simulink model "Final_lateral__"  (R2021a)
settings: Solver=VariableStepAuto  StartTime=0.0  StopTime=20  RelTol=1e-3
values from neighbouring files (symbols this model uses):
  A = [-2.3817 0 -1.0019 2.1827; -21.063 -16.055 0.87229 0; 24.512 -16.651 -3.5379 0; 0 1.0026 -0.029766 0]    [lateral_parameters.m]
  B = [0 -0.24719; -36.263 -688.44; -0.6725 -67.983; 0 0]    [lateral_parameters.m]
  B1 = [0.0869 0;4.424 1.184; 0 -1; -2.148 0.021]    [lateral_parameters.m]
  K = [K_hat(:,1) K_hat(:,2) K_hat(:,3) K_hat(:,4)]    [lateral_parameters.m]
  ki = [K_hat(:,5) K_hat(:,6)]    [lateral_parameters.m]
libraries: dspsrcs4 x1
settings Model: Creator=Lenovo  LastModifiedBy=Lenovo

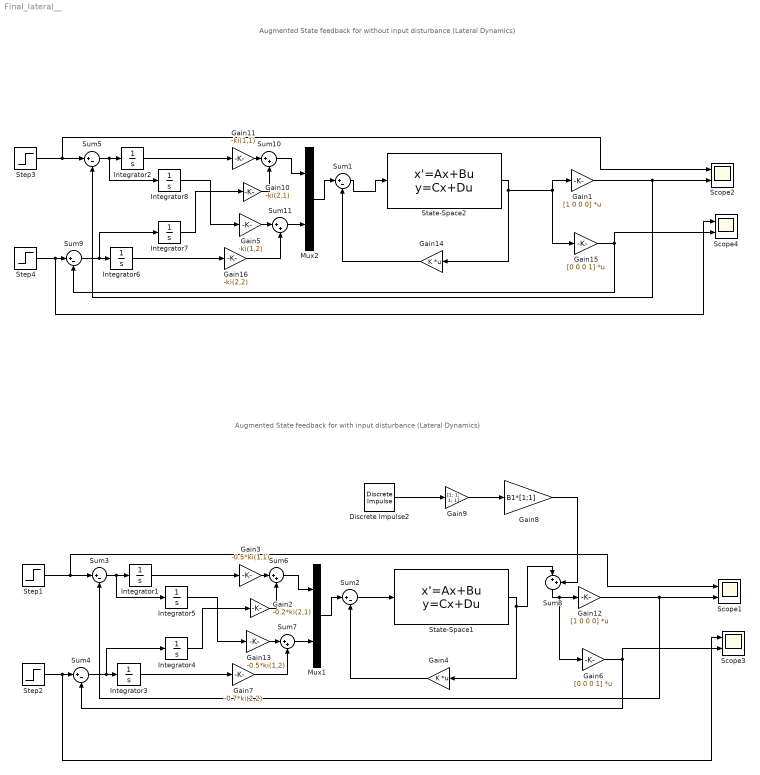
== system Final_lateral__ ==
  note: Augmented State feedback for without input disturbance (Lateral Dynamics)
  note: Augmented State feedback for with input disturbance (Lateral Dynamics)
  Discrete Impulse2 : dspsrcs4/Discrete  Impulse  Delay=0  SampleTime=1  FrameSample=1  OutputFrames=off  dataType=double  isSigned=on  wordLen=16  udDataType=sfix(16)  fracBitsMode=Best precision  numFracBits=15  OutDataTypeStr=double  LastOutDataTypeStr=double
  Gain1 : Gain  Gain=[1 0 0 0]  Multiplication=Matrix(K*u) (u vector)
  Gain10 : Gain  Gain=-ki(2,1)
  Gain11 : Gain  Gain=-ki(1,1)
  Gain12 : Gain  Gain=[1 0 0 0]  Multiplication=Matrix(K*u) (u vector)
  Gain13 : Gain  Gain=-0.5*ki(1,2)
  Gain14 : Gain  Gain=K  Multiplication=Matrix(K*u)
  Gain15 : Gain  Gain=[0 0 0 1]  Multiplication=Matrix(K*u) (u vector)
  Gain16 : Gain  Gain=-ki(2,2)
  Gain2 : Gain  Gain=-0.2*ki(2,1)
  Gain3 : Gain  Gain=-0.5*ki(1,1)
  Gain4 : Gain  Gain=K  Multiplication=Matrix(K*u)
  Gain5 : Gain  Gain=-ki(1,2)
  Gain6 : Gain  Gain=[0 0 0 1]  Multiplication=Matrix(K*u) (u vector)
  Gain7 : Gain  Gain=-0.7*ki(2,2)
  Gain8 : Gain  Gain=B1*[1;1]
  Gain9 : Gain  Gain=[1; 1; 1; 1]
  Integrator{1..8} (8 alike) : Integrator
  Mux1 : Mux  Inputs=2
  Mux2 : Mux  Inputs=2
  Scope{1..4} (4 alike) : Scope  NumInputPorts=2
  State-Space1 : StateSpace  A=A  B=B  C=eye(4)  D=zeros(4,2)  InitialCondition=0
  State-Space2 : StateSpace  A=A  B=B  C=eye(4)  D=zeros(4,2)  InitialCondition=0
  Step{1..4} (4 alike) : Step  Time=0  After=0.2  SampleTime=0
  Sum{1..5,9} (6 alike) : Sum  Inputs=|+-
  Sum{6..8,10..11} (5 alike) : Sum  Inputs=|++
  wires:
  Gain9/1 -> Gain8/1
  Discrete Impulse2/1 -> Gain9/1
  Sum2/1 -> State-Space1/1
  Integrator3/1 -> Gain7/1
  Gain6/1 -> Scope3/2, Sum4/2
  Sum3/1 -> Integrator5/1, Integrator1/1
  Step2/1 -> Scope3/1, Sum4/1
  Step1/1 -> Sum3/1, Scope1/1
  State-Space1/1 -> Sum8/1, Gain4/1
  Gain12/1 -> Scope1/2, Sum3/2
  Integrator1/1 -> Gain3/1
  Sum4/1 -> Integrator4/1, Integrator3/1
  Gain4/1 -> Sum2/2
  Gain3/1 -> Sum6/1
  Sum6/1 -> Mux1/1
  Gain7/1 -> Sum7/2
  Sum7/1 -> Mux1/2
  Integrator5/1 -> Gain13/1
  Gain13/1 -> Sum7/1
  Gain2/1 -> Sum6/2
  Integrator4/1 -> Gain2/1
  Mux1/1 -> Sum2/1
  Sum8/1 -> Gain6/1, Gain12/1
  Gain8/1 -> Sum8/2
  Step3/1 -> Sum5/1, Scope2/1
  Step4/1 -> Scope4/1, Sum9/1
  Integrator6/1 -> Gain16/1
  Sum1/1 -> State-Space2/1
  Mux2/1 -> Sum1/1
  State-Space2/1 -> Gain1/1, Gain15/1, Gain14/1
  Sum11/1 -> Mux2/2
  Sum5/1 -> Integrator8/1, Integrator2/1
  Gain1/1 -> Scope2/2, Sum5/2
  Sum9/1 -> Integrator7/1, Integrator6/1
  Integrator2/1 -> Gain11/1
  Gain5/1 -> Sum11/1
  Integrator7/1 -> Gain10/1
  Gain15/1 -> Scope4/2, Sum9/2
  Gain10/1 -> Sum10/2
  Integrator8/1 -> Gain5/1
  Gain11/1 -> Sum10/1
  Sum10/1 -> Mux2/1
  Gain16/1 -> Sum11/2
  Gain14/1 -> Sum1/2
